simulink model "cv_simple"  (R2019a)
settings: Solver=ode1  StartTime=0.0  StopTime=50  FixedStep=0.01  RelTol=1e-3
libraries: simulink x1, mpclib x1
settings Model: Creator=alexh  LastModifiedBy=alexh
settings DebuggingCC: UnderSpecifiedDimensionMsg=warning

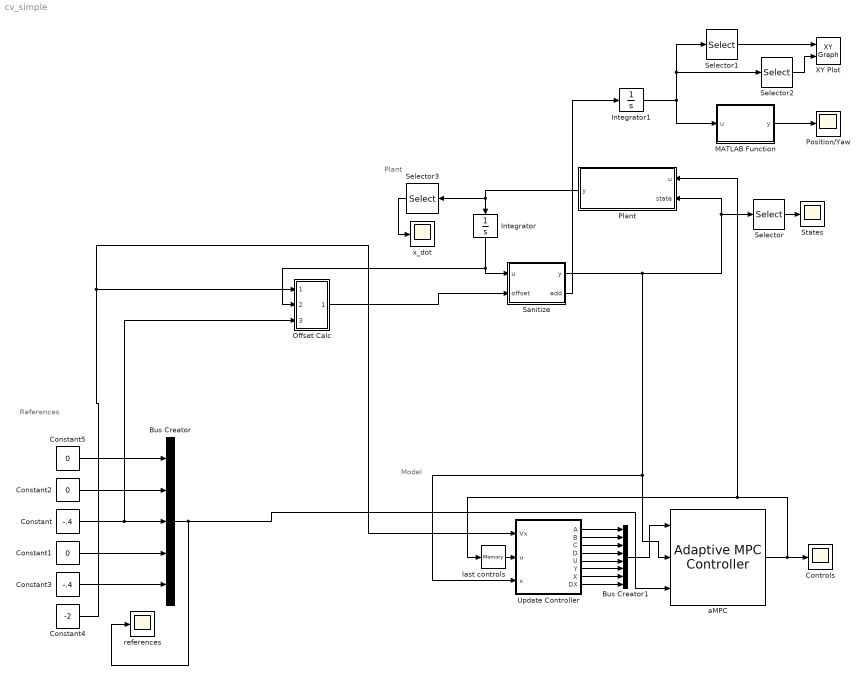
== system cv_simple ==
  note: Plant
  note: References
  note: Model
  Bus Creator : BusCreator  Inputs=5
  Bus Creator1 : BusCreator  Inputs=8
  Constant : Constant  Value=-.4
  Constant1 : Constant  Value=0
  Constant2 : Constant  Value=0
  Constant3 : Constant  Value=-.4
  Constant4 : Constant  Value=-2
  Constant5 : Constant  Value=0
  Controls : Scope
  Integrator : Integrator
  Integrator1 : Integrator
  MATLAB Function : MATLAB Function  TreatAsAtomicUnit=on
  Offset Calc : Subsystem
  Plant : MATLAB Function  TreatAsAtomicUnit=on
  Position/Yaw : Scope
  Sanitize : MATLAB Function  TreatAsAtomicUnit=on
  Selector : Selector  InputPortWidth=5  IndexOptions=Index vector (dialog)  Indices=[1 2 3 4]  OutputSizes=1
  Selector1 : Selector  InputPortWidth=3  IndexOptions=Index vector (dialog)  Indices=[1]  OutputSizes=1
  Selector2 : Selector  InputPortWidth=3  IndexOptions=Index vector (dialog)  Indices=[2]  OutputSizes=1
  Selector3 : Selector  InputPortWidth=5  IndexOptions=Index vector (dialog)  Indices=[1 2 3 4]  OutputSizes=1
  States : Scope
  Update Controller : MATLAB Function  TreatAsAtomicUnit=on
  XY Plot : simulink/Sinks/XY Graph  xmin=-20  xmax=20  ymin=-20  ymax=20  st=-1
  aMPC : mpclib/Adaptive MPC Controller  SCDEnableBlockLinearizationSpecification=on  mpcobj=mpc2  enable_value=0  updateMPCinCallerWorkspace=on  md_inport=off  mv_inport=off  uref_inport=off  return_cost=off  return_mvseq=off  return_qpstatus=off  return_xseq=off  return_state=off  return_ovseq=off  state_inport=off  isltv_plant=off  umin_inport=off  umax_inport=off  ymin_inport=off  ymax_inport=off  cc_inport=off  ywt_inport=off  uwt_inport=off  duwt_inport=off  rhoeps_inport=off  pm_inport=off  MaximumP=10  HorizonChoice=FixedHorizon  BlockDataType=double  SampleTimeInherited=off  switch_inport=off
      settings: SourceProductName=MATLAB Runtime - Model Predictive Control Toolbox Addin  SourceProductBaseCode=Missing
  last controls : Memory
  references : Scope
  x_dot : Scope
  wires:
  Constant/1 -> Bus Creator/3, Offset Calc/3(In3)
  Constant1/1 -> Bus Creator/4
  Bus Creator/1 -> aMPC/3, references/1
  aMPC/1 -> Plant/1(u), last controls/1, Controls/1
  Plant/1(y) -> Integrator/1, Selector3/1
  Integrator/1 -> Sanitize/1(u), Offset Calc/2(In2)
  Selector/1 -> States/1
  Constant2/1 -> Bus Creator/2
  Sanitize/1(y) -> Selector/1, Plant/2(state), Update Controller/3(x), aMPC/2
  Integrator1/1 -> Selector1/1, Selector2/1, MATLAB Function/1(u)
  Selector1/1 -> XY Plot/1
  Selector2/1 -> XY Plot/2
  Sanitize/2(add) -> Integrator1/1
  Constant3/1 -> Bus Creator/5
  Constant4/1 -> Update Controller/1(Vx), Offset Calc/1(In1)
  Update Controller/1(A) -> Bus Creator1/1
  Update Controller/2(B) -> Bus Creator1/2
  Update Controller/3(C) -> Bus Creator1/3
  Update Controller/4(D) -> Bus Creator1/4
  Update Controller/5(U) -> Bus Creator1/5
  Update Controller/6(Y) -> Bus Creator1/6
  Update Controller/7(X) -> Bus Creator1/7
  Update Controller/8(DX) -> Bus Creator1/8
  Bus Creator1/1 -> aMPC/1
  last controls/1 -> Update Controller/2(u)
  Constant5/1 -> Bus Creator/1
  Offset Calc/1(Out1) -> Sanitize/2(offset)
  MATLAB Function/1(y) -> Position/Yaw/1
  Selector3/1 -> x_dot/1

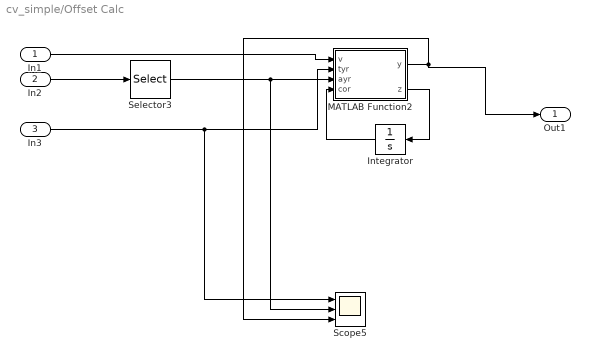
== system cv_simple/Offset Calc ==
  In1 : Inport
  In2 : Inport  Port=2
  In3 : Inport  Port=3
  Integrator : Integrator  InitialCondition=2
  MATLAB Function2 : MATLAB Function  TreatAsAtomicUnit=on
  Scope5 : Scope  NumInputPorts=3
  Selector3 : Selector  InputPortWidth=5  IndexOptions=Index vector (dialog)  Indices=[3]  OutputSizes=1
  Out1 : Outport
  wires:
  In3/1 -> MATLAB Function2/2(tyr), Scope5/1
  MATLAB Function2/1(y) -> Out1/1, Scope5/3
  Selector3/1 -> MATLAB Function2/3(ayr), Scope5/2
  In2/1 -> Selector3/1
  MATLAB Function2/2(z) -> Integrator/1
  In1/1 -> MATLAB Function2/1(v)
  Integrator/1 -> MATLAB Function2/4(cor)

== matlab function cv_simple/Sanitize ==
  data: u input; y output; add output; offset input
function [y, add]= fcn(u, offset)

u(1) = offset;
y = u;

Vx = 2;
add = [cos(y(2))*Vx; sin(y(2))*Vx; y(3)];

== matlab function cv_simple/Plant ==
  data: u input; y output; state input
function y = fcn(u, state)

m = 30;     % Mass
lf = 0.7;   % Distance mass center/front wheel
lr = 0.3;   % Distance mass center/rear wheel
cf = 3000;   % Cornering Stiffness front
cr = 3000;   % Cornering Stiffness rear
iz = 100;   % Yaw Moment of Innertia

Vx = 2.0;

% Continuous-time model
Ac = [0, 0, -Vx, 0, +Vx;
      0, 0, 1, 0, 0;
      0, 0, -(cr*lr^2+cf*lf^2)/(iz*Vx), -(cr*lr-cf*lf)/iz, 0;
      0, 0, 1-(cr*lr-cf*lf)/(m*Vx^2), -(cf+cr)/(m*Vx), 0;
      0, 0, 0, 0, -1];
   
Bc = [0, 0, cf*lf/iz, -cf/(m*Vx), 0;
      0, 0, 0, 0, -1]';

y = Ac*state + Bc*u;

== matlab function cv_simple/Offset Calc/MATLAB Function2 ==
  data: v input; tyr input; ayr input; y output; z output; cor input
function [y, z]= fcn(v, tyr, ayr, cor)

correction_angle = (ayr-tyr)+cor;

y = correction_angle*v;
z = (ayr-tyr);

== matlab function cv_simple/Update Controller ==
  data: Vx input; u input; A output; x input; B output; C output; D output; U output; Y output; X output; DX output
function [A,B,C,D,U,Y,X,DX] = fcn(Vx,u,x)

m = 30;     % Mass
lf = 0.7;   % Distance mass center/front wheel
lr = 0.3;   % Distance mass center/rear wheel
cf = 3000;   % Cornering Stiffness front
cr = 3000;   % Cornering Stiffness rear
iz = 100;   % Yaw Moment of Innertia

Ts = 0.01;

if (Vx<0.1)
       Vx = 0.1;
end

% Continuous-time model
Ac = [1, 0, -Vx, 0, +Vx;
       0, 0, 1, 0, 0;
       0, 0, -(cr*lr^2+cf*lf^2)/(iz*Vx), -(cr*lr-cf*lf)/iz, 0;
       0, 0, 1-(cr*lr-cf*lf)/(m*Vx^2), -(cf+cr)/(m*Vx), 0;
       0, 0, 0, 0, -.99];
       
Bc = [0, 0, cf*lf/iz, -cf/(m*Vx), 0;
      0, 0, 0, 0, -.99]';
 
% Position, Yaw, Speed
Cc = eye(5);
    
Dc = zeros(5, 2);

% Generate discrete-time model
nx = size(Ac,1);
nu = size(Bc,2);
M = expm([[Ac Bc]*Ts; zeros(nu, nx+nu)]);
A = M(1:nx, 1:nx);
B = M(1:nx, nx+1:nx+nu);
C = Cc;
D = Dc;

X = x';
U = u';
Y = (C*x + D*u)';
DX = (A*x + B*u - x)';

== matlab function cv_simple/MATLAB Function ==
  data: u input; y output
function y = fcn(u)

yaw_off = u(3)-pi;
u(3) = mod(abs(yaw_off), 2*pi) * sign(yaw_off) + pi;

y = u;
